simulink model "LKA_Lenkung_CarMaker_DSR_kaskadiert"  (Simulink 7.9)
settings: Solver=ode23  StartTime=0.0  StopTime=tend  FixedStep=0.01  RelTol=1e-3
undefined symbols (not defined in the file or in its folder): pin
libraries: library x6
settings Model: Creator=Georg  LastModifiedBy=georgnestlinger
settings DebuggingCC: FcnCallInpInsideContextMsg=Use local settings  StrictBusMsg=Warning
settings GRTTargetCC: CombineOutputUpdateFcns=off  GRTInterface=on

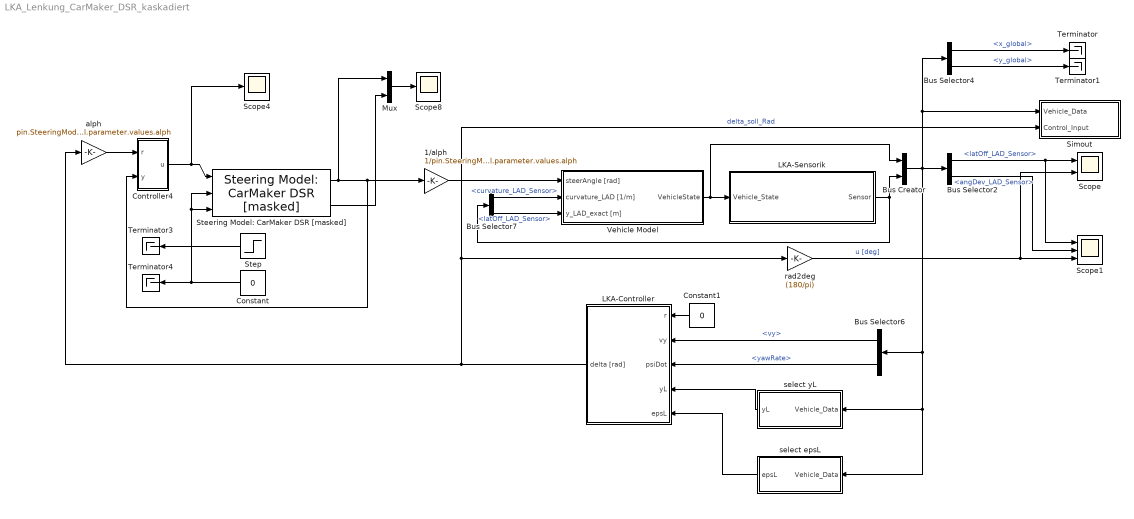
== system LKA_Lenkung_CarMaker_DSR_kaskadiert ==
  1/alph : Gain  Gain=1/pin.SteeringModel.parameter.values.alph
  Bus Creator : BusCreator  Inputs=2
  Bus Selector2 : BusSelector  OutputSignals=Sensor.latOff_LAD_Sensor,Sensor.angDev_LAD_Sensor
  Bus Selector4 : BusSelector  OutputSignals=VehicleState.x_global,VehicleState.y_global
  Bus Selector6 : BusSelector  OutputSignals=VehicleState.vy,VehicleState.yawRate
  Bus Selector7 : BusSelector  OutputSignals=curvature_LAD_Sensor,latOff_LAD_Sensor
  Constant : Constant  Value=0
  Constant1 : Constant  Value=0
  Controller4 : Subsystem
  LKA-Controller : Subsystem  BlockChoice=LQR_2int
      settings: AttributesFormatString=%<BlockChoice>  TemplateBlock=library/LKA-Controller/LKA-Controller  MemberBlocks=AlgSynth,FKL,LQR,LQR_2int,ZR,ZR_2int
  LKA-Sensorik : Subsystem  BlockChoice=Videosensorik
      settings: AttributesFormatString=%<BlockChoice>  TemplateBlock=library/LKA-Sensorik/LKA-Sensorik  MemberBlocks=Videosensorik
  Mux : Mux  Inputs=2
  Scope : Scope  NumInputPorts=2
      settings: TimeRange=12.76  YMin=-0.0018~1.07115  YMax=-2.1684e-019~1.0721
  Scope1 : Scope  NumInputPorts=3
      settings: TimeRange=20  YMin=-0.001~0.0215~0.915  YMax=0.003~0.0235~0.985
  Scope4 : Scope
      settings: YMin=-2.25e-007  YMax=3.5e-007  SaveName=ScopeData4
  Scope8 : Scope
      settings: TimeRange=12.76  YMin=-0.8  YMax=1.5  SaveName=ScopeData9
  Simout : Subsystem
  Steering Model: CarMaker DSR [masked] : library/Steering Models/Steering Model: CarMaker DSR [masked]  d_rot=pin.SteeringModel.parameter.values.drot  d_rack=pin.SteeringModel.parameter.values.drack  i=pin.SteeringModel.parameter.values.iHR  I_rot=pin.SteeringModel.parameter.values.J  m_left=pin.SteeringModel.parameter.values.mL  m_right=pin.SteeringModel.parameter.values.mR  m_rack=pin.SteeringModel.parameter.values.mr  V=pin.SteeringModel.parameter.values.V
  Step : Step  Time=10  SampleTime=0
  Terminator{,1,3..4} (4 alike) : Terminator
  Vehicle Model : Subsystem
  alph : Gain  Gain=pin.SteeringModel.parameter.values.alph
  "rad2deg " : Gain  Gain=(180/pi)
  select epsL : Subsystem  BlockChoice=epsL_exactMdl
      settings: AttributesFormatString=%<BlockChoice>  TemplateBlock=library/LKA-Sensorik/select epsL  MemberBlocks=epsL_Sensor,epsL_exactMdl,epsL_linMdl
  select yL : Subsystem  BlockChoice=yL_Sensor
      settings: AttributesFormatString=%<BlockChoice>  TemplateBlock=library/LKA-Sensorik/select yL  MemberBlocks=yL_Sensor,yL_exactMdl,yL_linMdl
  wires:
  Bus Selector4/1 -> Terminator/1  "<x_global>"
  Bus Selector4/2 -> Terminator1/1  "<y_global>"
  LKA-Controller/1(delta [rad]) -> alph/1, "rad2deg "/1, Simout/2(Control_Input)  "delta_soll_Rad"
  Bus Selector2/1 -> Scope/1, Scope1/1  "<latOff_LAD_Sensor>"
  Bus Selector2/2 -> Scope1/2  "<angDev_LAD_Sensor>"
  "rad2deg "/1 -> Scope/2, Scope1/3  "u [deg]"
  Controller4/1(u) -> Scope4/1, Steering Model: CarMaker DSR [masked]/1
  Steering Model: CarMaker DSR [masked]/1 -> Controller4/2(y), 1/alph/1, Mux/1
  alph/1 -> Controller4/1(r)
  Mux/1 -> Scope8/1
  Step/1 -> Terminator3/1
  Constant/1 -> Terminator4/1, Steering Model: CarMaker DSR [masked]/3, Steering Model: CarMaker DSR [masked]/2
  Constant1/1 -> LKA-Controller/1(r)
  Bus Selector6/1 -> LKA-Controller/2(vy)  "<vy>"
  Bus Selector6/2 -> LKA-Controller/3(psiDot)  "<yawRate>"
  select yL/1(yL) -> LKA-Controller/4(yL)
  select epsL/1(epsL) -> LKA-Controller/5(epsL)
  LKA-Sensorik/1(Sensor) -> Bus Creator/2, Bus Selector7/1
  Vehicle Model/1(VehicleState) -> Bus Creator/1, LKA-Sensorik/1(Vehicle_State)
  1/alph/1 -> Vehicle Model/1(steerAngle [rad])
  Bus Selector7/2 -> Vehicle Model/3(y_LAD_exact [m])  "<latOff_LAD_Sensor>"
  Bus Selector7/1 -> Vehicle Model/2(curvature_LAD [1/m])  "<curvature_LAD_Sensor>"
  Bus Creator/1 -> Bus Selector6/1, select yL/1(Vehicle_Data), select epsL/1(Vehicle_Data), Bus Selector2/1, Bus Selector4/1, Simout/1(Vehicle_Data)
  Steering Model: CarMaker DSR [masked]/2 -> Mux/2

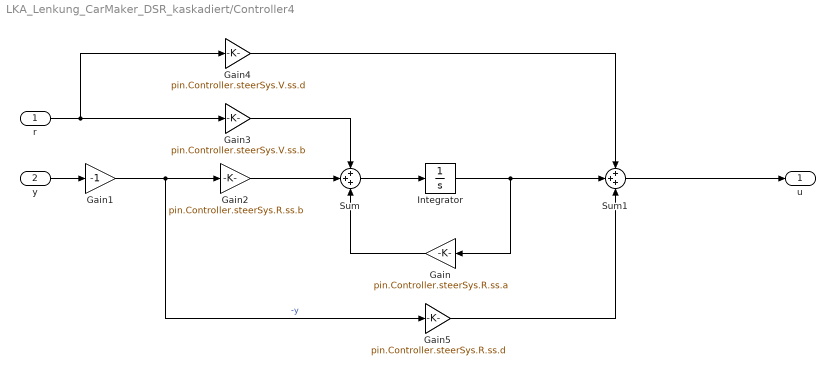
== system LKA_Lenkung_CarMaker_DSR_kaskadiert/Controller4 ==
  r : Inport
  y : Inport  Port=2
  Gain : Gain  Gain=pin.Controller.steerSys.R.ss.a
  Gain1 : Gain  Gain=-1
  Gain2 : Gain  Gain=pin.Controller.steerSys.R.ss.b
  Gain3 : Gain  Gain=pin.Controller.steerSys.V.ss.b
  Gain4 : Gain  Gain=pin.Controller.steerSys.V.ss.d
  Gain5 : Gain  Gain=pin.Controller.steerSys.R.ss.d
  Integrator : Integrator
  Sum : Sum  Inputs=+++
  Sum1 : Sum  Inputs=+++
  u : Outport
  wires:
  Sum1/1 -> u/1
  Gain5/1 -> Sum1/3
  Gain4/1 -> Sum1/1
  Integrator/1 -> Sum1/2, Gain/1
  Gain3/1 -> Sum/1
  r/1 -> Gain4/1, Gain3/1
  Gain2/1 -> Sum/2
  Gain1/1 -> Gain5/1, Gain2/1  "-y"
  y/1 -> Gain1/1
  Sum/1 -> Integrator/1
  Gain/1 -> Sum/3

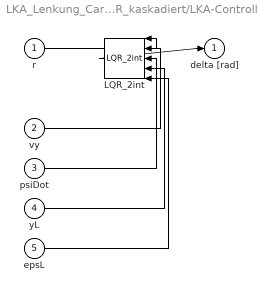
== system LKA_Lenkung_CarMaker_DSR_kaskadiert/LKA-Controller ==
  r : Inport
  vy : Inport  Port=2
  psiDot : Inport  Port=3
  yL : Inport  Port=4
  epsL : Inport  Port=5
  LQR_2int : library/LKA-Controller/LQR_2int
  delta [rad] : Outport
  wires:
  r/1 -> LQR_2int/1
  vy/1 -> LQR_2int/2
  psiDot/1 -> LQR_2int/3
  yL/1 -> LQR_2int/4
  epsL/1 -> LQR_2int/5
  LQR_2int/1 -> delta [rad]/1

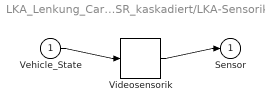
== system LKA_Lenkung_CarMaker_DSR_kaskadiert/LKA-Sensorik ==
  Vehicle_State : Inport
  Videosensorik : library/LKA-Sensorik/Videosensorik
  Sensor : Outport
  wires:
  Vehicle_State/1 -> Videosensorik/1
  Videosensorik/1 -> Sensor/1

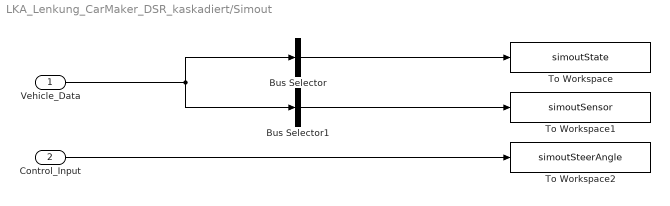
== system LKA_Lenkung_CarMaker_DSR_kaskadiert/Simout ==
  Vehicle_Data : Inport
  Control_Input : Inport  Port=2
  Bus Selector : BusSelector  OutputSignals=VehicleState  OutputAsBus=on
  Bus Selector1 : BusSelector  OutputSignals=Sensor  OutputAsBus=on
  To Workspace : ToWorkspace  VariableName=simoutState  SampleTime=-1  SaveFormat=Structure With Time
  To Workspace1 : ToWorkspace  VariableName=simoutSensor  SampleTime=-1  SaveFormat=Structure With Time
  To Workspace2 : ToWorkspace  VariableName=simoutSteerAngle  SampleTime=-1  SaveFormat=Structure With Time
  wires:
  Vehicle_Data/1 -> Bus Selector1/1, Bus Selector/1
  Control_Input/1 -> To Workspace2/1
  Bus Selector/1 -> To Workspace/1
  Bus Selector1/1 -> To Workspace1/1

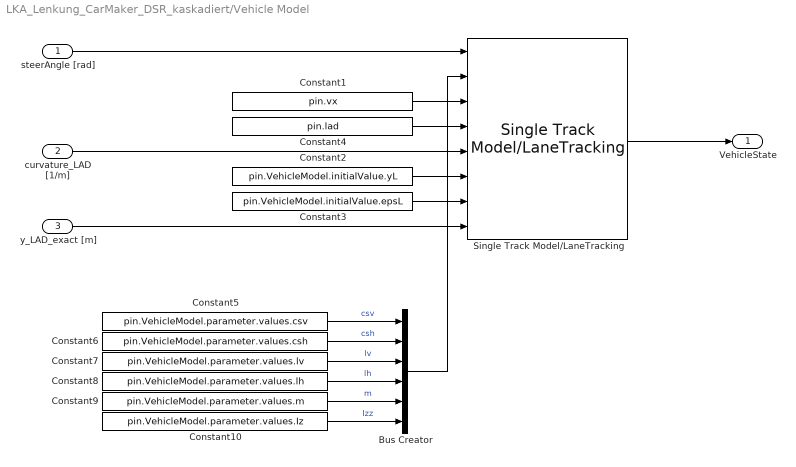
== system LKA_Lenkung_CarMaker_DSR_kaskadiert/Vehicle Model ==
  steerAngle [rad] : Inport
  curvature_LAD [1/m] : Inport  Port=2
  y_LAD_exact [m] : Inport  Port=3
  Bus Creator : BusCreator  Inputs=6
  Constant1 : Constant  Value=pin.vx
  Constant10 : Constant  Value=pin.VehicleModel.parameter.values.Iz
  Constant2 : Constant  Value=pin.VehicleModel.initialValue.yL
  Constant3 : Constant  Value=pin.VehicleModel.initialValue.epsL
  Constant4 : Constant  Value=pin.lad
  Constant5 : Constant  Value=pin.VehicleModel.parameter.values.csv
  Constant6 : Constant  Value=pin.VehicleModel.parameter.values.csh
  Constant7 : Constant  Value=pin.VehicleModel.parameter.values.lv
  Constant8 : Constant  Value=pin.VehicleModel.parameter.values.lh
  Constant9 : Constant  Value=pin.VehicleModel.parameter.values.m
  Single Track Model/LaneTracking : library/Vehicle Models/Single Track Model//LaneTracking
  VehicleState : Outport
  wires:
  Single Track Model/LaneTracking/1 -> VehicleState/1
  Constant2/1 -> Single Track Model/LaneTracking/6
  Constant3/1 -> Single Track Model/LaneTracking/7
  Constant1/1 -> Single Track Model/LaneTracking/3
  Constant4/1 -> Single Track Model/LaneTracking/4
  steerAngle [rad]/1 -> Single Track Model/LaneTracking/1
  curvature_LAD [1/m]/1 -> Single Track Model/LaneTracking/5
  y_LAD_exact [m]/1 -> Single Track Model/LaneTracking/8
  Constant5/1 -> Bus Creator/1  "csv"
  Constant6/1 -> Bus Creator/2  "csh"
  Constant7/1 -> Bus Creator/3  "lv"
  Constant8/1 -> Bus Creator/4  "lh"
  Constant9/1 -> Bus Creator/5  "m"
  Constant10/1 -> Bus Creator/6  "Izz"
  Bus Creator/1 -> Single Track Model/LaneTracking/2

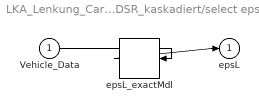
== system LKA_Lenkung_CarMaker_DSR_kaskadiert/select epsL ==
  Vehicle_Data : Inport
  epsL_exactMdl : library/LKA-Sensorik/epsL_exactMdl
  epsL : Outport
  wires:
  Vehicle_Data/1 -> epsL_exactMdl/1
  epsL_exactMdl/1 -> epsL/1

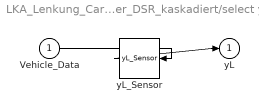
== system LKA_Lenkung_CarMaker_DSR_kaskadiert/select yL ==
  Vehicle_Data : Inport
  yL_Sensor : library/LKA-Sensorik/yL_Sensor
  yL : Outport
  wires:
  Vehicle_Data/1 -> yL_Sensor/1
  yL_Sensor/1 -> yL/1
